simulink model "sim_red_at_lgr"  (R2020b)
settings: Solver=VariableStepAuto  StartTime=0.0  StopTime=100  RelTol=1e-3
values from neighbouring files (symbols this model uses):
  den = conv(den,[1 2])    [lgr_atraso.m]
  k = 1.05    [lgr_atraso.m]    (also in lgr_atraso_adelanto.m = 1/div)
  p = 0.005    [lgr_atraso.m]
  z = p*10    (= 0.05)    [lgr_atraso.m]
libraries: simulink x2
settings Model: Creator=Acer  LastModifiedBy=Acer

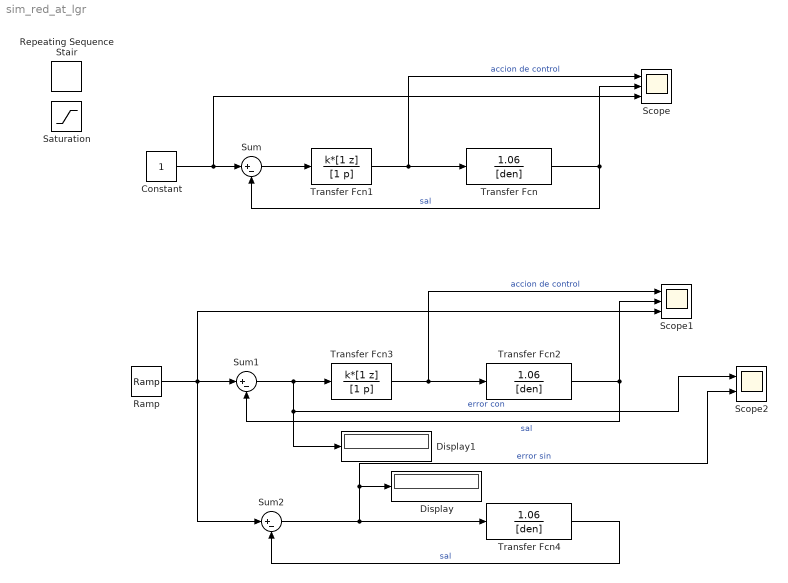
== system sim_red_at_lgr ==
  Constant : Constant  SampleTime=6
  Display : Display
  Display1 : Display
  Ramp : simulink/Sources/Ramp  slope=1  start=0  InitialOutput=0
  Repeating Sequence Stair : simulink/Sources/Repeating Sequence Stair  OutValues=[1 -0.5 2 5 -2.5].'  tsamp=6  OutMin=[]  OutMax=[]  OutDataTypeStr=double  OutputDataTypeScalingMode=double  OutDataType=fixdt(0,8)  ConRadixGroup=Best Precision: Vector-wise  OutScaling=2^-12
  Saturation : Saturate  UpperLimit=13  LowerLimit=-13
  Scope : Scope  NumInputPorts=3
  Scope1 : Scope  NumInputPorts=3
  Scope2 : Scope  NumInputPorts=2
  Sum : Sum  Inputs=|+-
  Sum1 : Sum  Inputs=|+-
  Sum2 : Sum  Inputs=|+-
  Transfer Fcn : TransferFcn  Numerator=[1.06]  Denominator=[den]
  Transfer Fcn1 : TransferFcn  Numerator=k*[1 z]  Denominator=[1 p]
  Transfer Fcn2 : TransferFcn  Numerator=[1.06]  Denominator=[den]
  Transfer Fcn3 : TransferFcn  Numerator=k*[1 z]  Denominator=[1 p]
  Transfer Fcn4 : TransferFcn  Numerator=[1.06]  Denominator=[den]
  wires:
  Transfer Fcn1/1 -> Transfer Fcn/1, Scope/1  "accion de control"
  Transfer Fcn/1 -> Scope/2, Sum/2  "sal"
  Sum/1 -> Transfer Fcn1/1
  Constant/1 -> Scope/3, Sum/1
  Transfer Fcn2/1 -> Scope1/2, Sum1/2  "sal"
  Transfer Fcn3/1 -> Transfer Fcn2/1, Scope1/1  "accion de control"
  Sum1/1 -> Display1/1, Scope2/1, Transfer Fcn3/1  "error con"
  Sum2/1 -> Display/1, Scope2/2, Transfer Fcn4/1  "error sin"
  Transfer Fcn4/1 -> Sum2/2  "sal"
  Ramp/1 -> Sum2/1, Scope1/3, Sum1/1
